simulink model "Three_Phase_Thristor_Rectifier"  (R2018b)
settings: Solver=VariableStepAuto  StartTime=0.0  StopTime=10.0  RelTol=1e-3
libraries: powerlib x13, powerlib_extras x1
settings Model: Creator=fkara  LastModifiedBy=fkara

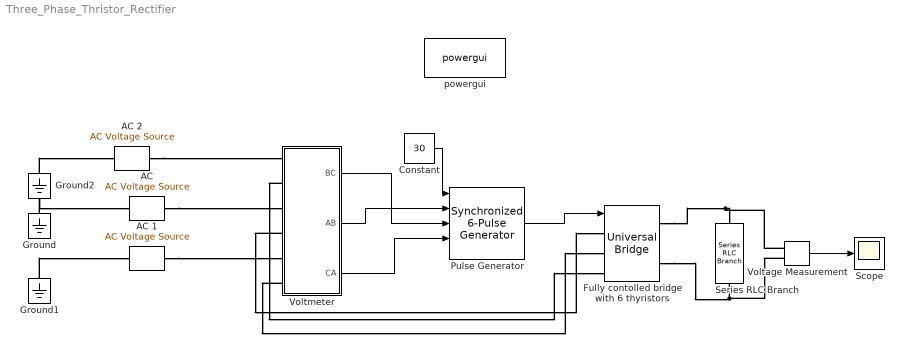
== system Three_Phase_Thristor_Rectifier ==
  "AC " : powerlib/Electrical Sources/AC Voltage Source  Amplitude=400  Phase=0  Frequency=50  SampleTime=0  Measurements=Voltage  BusType=swing  Pref=10e3  Qref=0  Qmin=-inf  Qmax=+inf
      settings: SourceProductName=Simscape Electrical
  AC 1 : powerlib/Electrical Sources/AC Voltage Source  Amplitude=400  Phase=-120  Frequency=50  SampleTime=0  Measurements=Voltage  BusType=swing  Pref=10e3  Qref=0  Qmin=-inf  Qmax=+inf
      settings: SourceProductName=Simscape Electrical
  AC 2 : powerlib/Electrical Sources/AC Voltage Source  Amplitude=400  Phase=120  Frequency=50  SampleTime=0  Measurements=Voltage  BusType=swing  Pref=10e3  Qref=0  Qmin=-inf  Qmax=+inf
      settings: SourceProductName=Simscape Electrical
  Constant : Constant  Value=30
  Fully contolled bridge with 6 thyristors : powerlib/Power Electronics/Universal Bridge  Arms=3  SnubberResistance=1e5  SnubberCapacitance=inf  Device=Thyristors  Ron=1e-3  Lon=0  ForwardVoltages="[  0  0  ]"  ForwardVoltage=0  GTOparameters=[ 10e-6 , 20e-6 ]  IGBTparameters=[ 1e-6 , 2e-6 ]  Measurements=Device voltages  Measurements_2=None  converterType=Rectifier
      settings: SourceProductName=Simscape Electrical
  Ground : powerlib/Elements/Ground  LConnTagsString=a
      settings: SourceProductName=Simscape Electrical
  Ground1 : powerlib/Elements/Ground  LConnTagsString=a
      settings: SourceProductName=Simscape Electrical
  Ground2 : powerlib/Elements/Ground  LConnTagsString=a
      settings: SourceProductName=Simscape Electrical
  Pulse Generator : powerlib_extras/Control  Blocks/Synchronized 6-Pulse Generator  freq=50  pwidth=10  Double_Pulse=off
  Scope : Scope
  Series RLC Branch : powerlib/Elements/Series RLC Branch  LConnTagsString=__new0  RConnTagsString=__new0  BranchType=R  Resistance=100  Inductance=1e-3  SetiL0=off  InitialCurrent=0  Capacitance=1e-6  Setx0=off  InitialVoltage=0  Measurements=None
  Voltage Measurement : powerlib/Measurements/Voltage Measurement  PhasorSimulation=off  OutputType=Complex  PSBequivalent=0
  Voltmeter : Subsystem
  powergui : powerlib/powergui  Priority=1  SimulationMode=Discrete  SampleTime=50e-6  frequency=60  Iterations=50  frequencyindice=50  Pbase=100e6  ErrMax=1e-4  UnitsV=kV  UnitsW=MW  buscounter=0  FunctionMessages=off  echomessages=off  EnableUseOfTLC=off  CurrentSourceSwitches=off  DisableSnubberDevices=off  DisableRonSwitches=off  DisableVfSwitches=off  DisplayEquations=off  SolverType=Tustin/Backward Euler (TBE)  Interpol=off  ExternalGateDelay=off  methode=off  Ts=100  x0status=blocks  SPID=on  SwTol=0  HookPort=off  RestoreLinks=warning  ResistiveCurrentMeasurement=off  Frange=[0:2:500]  Ylog=off  Xlog=on  ShowGrid=off  save=off  variable=ZData  structure=0  ZoomFFT=off  StartTime=0.0  cycles=1  DisplayStyle=1  fundamental=60  FreqAxis=off  MaxFrequency=1000  frequencyindicesteady=1  RmsSteady=1  display=off
  wires:
  Constant/1 -> Pulse Generator/1
  Voltmeter/1(BC) -> Pulse Generator/3
  Voltmeter/2(AB) -> Pulse Generator/2
  Voltmeter/3(CA) -> Pulse Generator/4
  Pulse Generator/1 -> Fully contolled bridge with 6 thyristors/1
  Voltage Measurement/1 -> Scope/1
  connections:
  Ground/LConn1 -- "AC "/LConn1
  Ground1/LConn1 -- AC 1/LConn1
  Ground2/LConn1 -- AC 2/LConn1
  Fully contolled bridge with 6 thyristors/RConn1 -- Voltage Measurement/LConn1 -- Series RLC Branch/LConn1
  Fully contolled bridge with 6 thyristors/RConn2 -- Voltage Measurement/LConn2 -- Series RLC Branch/RConn1
  AC 2/RConn1 -- Voltmeter/LConn1
  "AC "/RConn1 -- Voltmeter/LConn3
  AC 1/RConn1 -- Voltmeter/LConn5
  Voltmeter/LConn2 -- Fully contolled bridge with 6 thyristors/LConn3
  Voltmeter/LConn4 -- Fully contolled bridge with 6 thyristors/LConn1
  Voltmeter/LConn6 -- Fully contolled bridge with 6 thyristors/LConn2

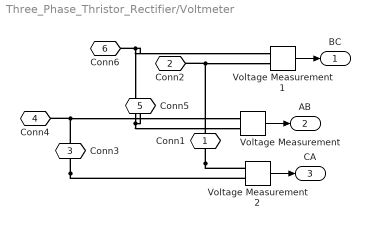
== system Three_Phase_Thristor_Rectifier/Voltmeter ==
  Voltage Measurement : powerlib/Measurements/Voltage Measurement  PhasorSimulation=off  OutputType=Complex  PSBequivalent=0
      settings: SourceProductName=Simscape Electrical
  Voltage Measurement1 : powerlib/Measurements/Voltage Measurement  PhasorSimulation=off  OutputType=Complex  PSBequivalent=0
      settings: SourceProductName=Simscape Electrical
  Voltage Measurement2 : powerlib/Measurements/Voltage Measurement  PhasorSimulation=off  OutputType=Complex  PSBequivalent=0
      settings: SourceProductName=Simscape Electrical
  Conn1 : PMIOPort  Side=Left
  Conn2 : PMIOPort  Port=2  Side=Left
  Conn3 : PMIOPort  Port=3  Side=Left
  Conn4 : PMIOPort  Port=4  Side=Left
  Conn5 : PMIOPort  Port=5  Side=Left
  Conn6 : PMIOPort  Port=6  Side=Left
  BC : Outport
  AB : Outport  Port=2
  CA : Outport  Port=3
  wires:
  Voltage Measurement1/1 -> BC/1
  Voltage Measurement/1 -> AB/1
  Voltage Measurement2/1 -> CA/1
  connections:
  Voltage Measurement2/LConn2 -- Conn4/RConn1 -- Voltage Measurement/LConn1 -- Conn3/RConn1
  Conn6/RConn1 -- Voltage Measurement1/LConn1 -- Voltage Measurement/LConn2 -- Conn5/RConn1
  Voltage Measurement2/LConn1 -- Conn2/RConn1 -- Voltage Measurement1/LConn2 -- Conn1/RConn1
